simulink model "untitled1"  (R2019b)
settings: Solver=VariableStepAuto  StartTime=0.0  StopTime=10.0  RelTol=1e-3
undefined symbols (not defined in the file or in its folder): sigbuilder_block
libraries: simulink x5
settings Model: Creator=YJR  LastModifiedBy=YJR

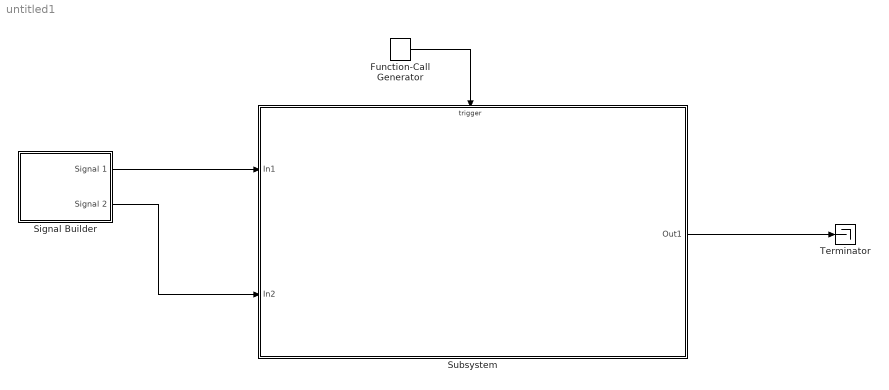
== system untitled1 ==
  Function-Call Generator : simulink/Ports & Subsystems/Function-Call Generator  sample_time=0.01  numberOfIterations=1
  Signal Builder : Subsystem  Tag=STV Subsys  LoadFcn=sigbuilder_block('load');  StartFcn=sigbuilder_block('start');  StopFcn=sigbuilder_block('stop');  ClipboardFcn=sigbuilder_block('clipboard');  mask(Sigbuilder block){tuvar=[0:10]}
      mask help: Simulink:masks:SigbuilderBlock_MD
      mask init:
      | if ~strcmp(get_param(bdroot(gcbh),'SimulationStatus'),'stopped') tuvar = sigbuilder_block('maskInit'); end
      settings: CopyFcn=sigbuilder_block('copy');  DeleteFcn=sigbuilder_block('delete');  ModelCloseFcn=sigbuilder_block('modelClose');  PreSaveFcn=sigbuilder_block('preSave');  PauseFcn=sigbuilder_block('pause');  ContinueFcn=sigbuilder_block('continue');  NameChangeFcn=sigbuilder_block('namechange');  OpenFcn=sigbuilder_block('open',[437.6 199.2 550.4 400 ]);  CloseFcn=sigbuilder_block('close');
      mask Display: plot(0, 0, 100, 100,[2, 2, 32, 32, 2], [68, 8, 8, 68, 68],[32, 2], [38, 38], [32, 19, 2],[53, 60, 44], [32, 17, 17, 2],[16, 16, 31, 31]);txt = getActiveGroup(gcbh);text(2, 100, txt,'verticalAlignment', 'top');
  Subsystem : Subsystem
  Terminator : Terminator
  wires:
  Function-Call Generator/1 -> Subsystem/Trigger
  Signal Builder/1(Signal 1) -> Subsystem/1(In1)
  Signal Builder/2(Signal 2) -> Subsystem/2(In2)
  Subsystem/1(Out1) -> Terminator/1

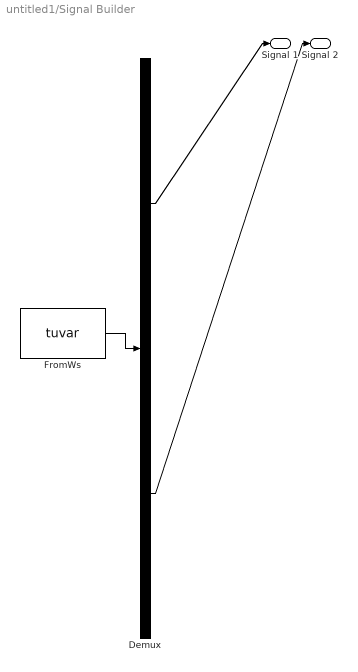
== system untitled1/Signal Builder ==
  Demux : Demux  Tag=STV Demux  Outputs=2
  FromWs : FromWorkspace  Tag=STV FromWs  VariableName=tuvar  SampleTime=0
      SigBuilderData=|
      | common.afterFinalStr = 'Extrapolate'
      | common.sampleTime = 0
      | dataSet.timeRange = [0 10]
      | dataSet.name = 'Group 1'
      | sbobj.Groups.Name = 'Group 1'
      | sbobj.Groups.Signals(1).Name = 'Signal 1'
      | sbobj.Groups.Signals(1).XData = [0 1.25 1.25 3.75 3.75 5 6.25 7.5 7.5 8.75 8.75 10]
      | sbobj.Groups.Signals(1).YData = [0 0 500 500 0 0 0 0 1 1 0 0]
      | sbobj.Groups.Signals(2).Name = 'Signal 2'
      | sbobj.Groups.Signals(2).XData = [0 0.74 0.74 5 5 6.36 6.36 8.06 8.06 10]
      | sbobj.Groups.Signals(2).YData = [1 1 0 0 1 1 0 0 1 1]
  Signal 1 : Outport  Tag=STV Outport
  Signal 2 : Outport  Tag=STV Outport  Port=2
  wires:
  FromWs/1 -> Demux/1
  Demux/1 -> Signal 1/1
  Demux/2 -> Signal 2/1

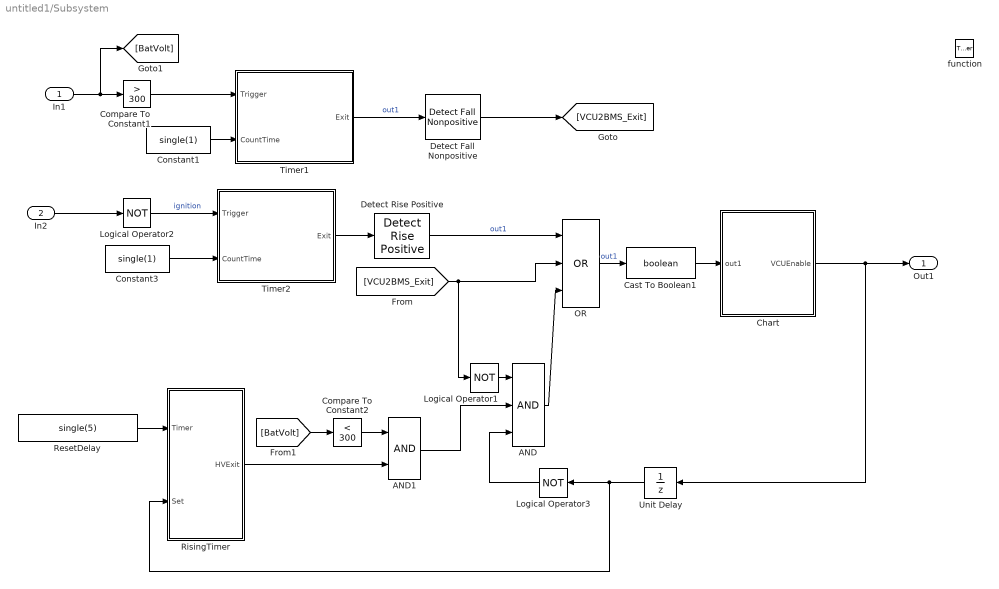
== system untitled1/Subsystem ==
  In1 : Inport
  In2 : Inport  Port=2
  function : TriggerPort  TriggerType=function-call  VariantControl=Variant
  AND : Logic  Inputs=3  AllPortsSameDT=off  OutDataTypeStr=boolean
  AND1 : Logic  AllPortsSameDT=off  OutDataTypeStr=boolean
  Cast To Boolean1 : DataTypeConversion  OutDataTypeStr=boolean
  Chart : Stateflow chart  BlockKeywords=__PRM__SERIALIZED__DATA__:Stateflow Chart,Stateflow Diagram  TreatAsAtomicUnit=on
  Compare To Constant1 : simulink/Logic and Bit Operations/Compare To Constant  relop=>  const=300  OutDataTypeStr=boolean
  Compare To Constant2 : simulink/Logic and Bit Operations/Compare To Constant  relop=<  const=300  OutDataTypeStr=boolean
  Constant1 : Constant  Value=single(1)
  Constant3 : Constant  Value=single(1)
  Detect Fall Nonpositive : simulink/Logic and Bit Operations/Detect Fall Nonpositive  vinit=1  OutDataTypeStr=boolean
      settings: SourceProductName=Simulink  SourceProductBaseCode=SL
  Detect Rise Positive : simulink/Logic and Bit Operations/Detect Rise Positive  vinit=0  OutDataTypeStr=boolean
  Logical Operator1 : Logic  Operator=NOT  AllPortsSameDT=off  OutDataTypeStr=boolean
  Logical Operator2 : Logic  Operator=NOT  AllPortsSameDT=off  OutDataTypeStr=boolean
  Logical Operator3 : Logic  Operator=NOT  AllPortsSameDT=off  OutDataTypeStr=boolean
  OR : Logic  Operator=OR  Inputs=3  AllPortsSameDT=off  OutDataTypeStr=boolean
  ResetDelay : Constant  Value=single(5)
  RisingTimer : Subsystem
  Timer1 : Stateflow chart  TreatAsAtomicUnit=on
  Timer2 : Stateflow chart  TreatAsAtomicUnit=on
  Unit Delay : UnitDelay  SampleTime=-1  HasFrameUpgradeWarning=on
  Out1 : Outport
  wires:
  In2/1 -> Logical Operator2/1
  [VCU2BMS_Exit] -> Logical Operator1/1, OR/2
  Timer1/1(Exit) -> Detect Fall Nonpositive/1  "out1"
  Cast To Boolean1/1 -> Chart/1(out1)
  Compare To Constant1/1 -> Timer1/1(Trigger)
  Detect Rise Positive/1 -> OR/1  "out1"
  AND/1 -> OR/3
  Unit Delay/1 -> Logical Operator3/1, RisingTimer/2(Set)
  ResetDelay/1 -> RisingTimer/1(Timer)
  Timer2/1(Exit) -> Detect Rise Positive/1
  OR/1 -> Cast To Boolean1/1  "out1"
  Constant3/1 -> Timer2/2(CountTime)
  RisingTimer/1(HVExit) -> AND1/2
  Constant1/1 -> Timer1/2(CountTime)
  Logical Operator1/1 -> AND/1
  Chart/1(VCUEnable) -> Out1/1, Unit Delay/1
  Logical Operator3/1 -> AND/3
  Compare To Constant2/1 -> AND1/1
  AND1/1 -> AND/2
  [BatVolt] -> Compare To Constant2/1
  Logical Operator2/1 -> Timer2/1(Trigger)  "ignition"
  Detect Fall Nonpositive/1 -> [VCU2BMS_Exit]
  In1/1 -> [BatVolt], Compare To Constant1/1

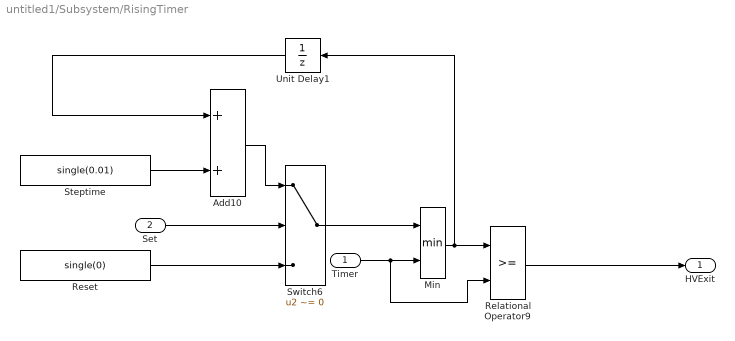
== system untitled1/Subsystem/RisingTimer ==
  Timer : Inport
  Set : Inport  Port=2
  Add10 : Sum
  Min : MinMax  Inputs=2
  Relational Operator9 : RelationalOperator  OutDataTypeStr=boolean  RndMeth=Simplest
  Reset : Constant  Value=single(0)
  Steptime : Constant  Value=single(0.01)
  Switch6 : Switch  Criteria=u2 ~= 0
  Unit Delay1 : UnitDelay  SampleTime=-1  HasFrameUpgradeWarning=on
  HVExit : Outport
  wires:
  Add10/1 -> Switch6/1
  Set/1 -> Switch6/2
  Min/1 -> Unit Delay1/1, Relational Operator9/1
  Unit Delay1/1 -> Add10/1
  Timer/1 -> Relational Operator9/2, Min/2
  Reset/1 -> Switch6/3
  Relational Operator9/1 -> HVExit/1
  Steptime/1 -> Add10/2
  Switch6/1 -> Min/1

== stateflow chart untitled1/Subsystem/Timer1 ==
  state Trigger
    en:
    x = x + 0.01;
    Exit=0;
  state Out
    en:
    Exit=1;
    x=0;
  state InterState
    en:
    x=0;
  Trigger -> Trigger [order 1] : [Trigger&&x<CountTime]
  Trigger -> Out [order 2] : [x>=CountTime]
  (default) -> Trigger
  Out -> Trigger : [~Trigger]
  InterState -> Trigger : [Trigger]
  Trigger -> InterState [order 3] : [x<CountTime&&~Trigger]
  data: Trigger input; CountTime input; Exit output; x local =0

== stateflow chart untitled1/Subsystem/Chart ==
  state STATEON
    state initstate
      en:
      VCUEnable=false;
    state ON
      en:
      VCUEnable=true;
    (default) -> initstate
    initstate -> ON : after(0.2,sec)[out1]
  state STATEOFF
    state initstate1
      en:
      VCUEnable=true;
    state OFF
      en:
      VCUEnable=false;
    (default) -> initstate1
    initstate1 -> OFF : after(0.2,sec)[out1]
  (default) -> STATEON
  ON -> STATEOFF
  OFF -> STATEON
  data: out1 input boolean; VCUEnable output boolean

== stateflow chart untitled1/Subsystem/Timer2 ==
  state Trigger
    en:
    x = x + 0.01;
    Exit=0;
  state Out
    en:
    Exit=1;
    x=0;
  state InterState
    en:
    x=0;
  Trigger -> Trigger [order 1] : [Trigger&&x<CountTime]
  Trigger -> Out [order 2] : [x>=CountTime]
  (default) -> Trigger
  Out -> Trigger : [~Trigger]
  InterState -> Trigger : [Trigger]
  Trigger -> InterState [order 3] : [x<CountTime&&~Trigger]
  data: Trigger input; CountTime input; Exit output; x local =0
